simulink model "traction_control_simulink"  (R2020b)
settings: Solver=VariableStepAuto  StartTime=0.0  StopTime=3  RelTol=1e-3
values from neighbouring files (symbols this model uses):
  N = 4    [run_simulation.m]
  Ts = 2e-3    (= 0.002)    [run_simulation.m]
  x0 = [1.4; 4.4]    [run_simulation.m]
libraries: pid_lib x1
settings Model: Creator=LAMES Workstation  LastModifiedBy=LAMES Workstation

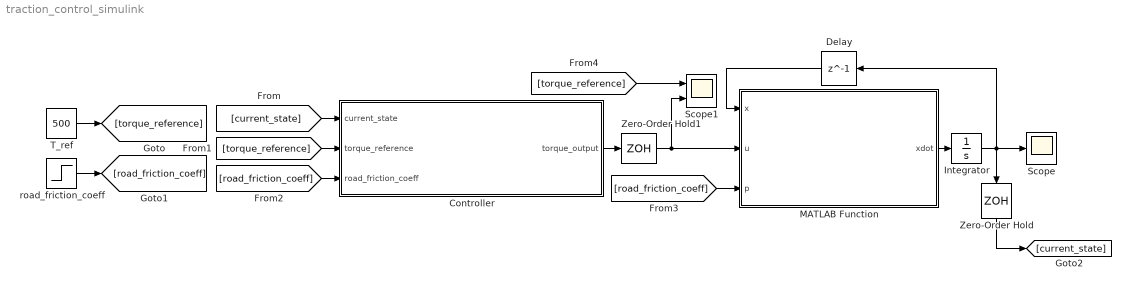
== system traction_control_simulink ==
  Controller : Subsystem  Variant=on
  Delay : Delay  DelayLength=1  InitialCondition=x0
  Integrator : Integrator  InitialCondition=x0
  MATLAB Function : MATLAB Function  TreatAsAtomicUnit=on
  Scope : Scope
  Scope1 : Scope  NumInputPorts=2
  T_ref : Constant  Value=500  SampleTime=Ts
  Zero-Order Hold : ZeroOrderHold  SampleTime=Ts
  Zero-Order Hold1 : ZeroOrderHold  SampleTime=Ts/100
  road_friction_coeff : Step  Time=0.5  Before=0.15  After=0.05  SampleTime=Ts
  wires:
  [road_friction_coeff] -> MATLAB Function/3(p)
  Delay/1 -> MATLAB Function/1(x)
  MATLAB Function/1(xdot) -> Integrator/1
  Zero-Order Hold/1 -> [current_state]
  Zero-Order Hold1/1 -> Scope1/2, MATLAB Function/2(u)
  Integrator/1 -> Zero-Order Hold/1, Scope/1, Delay/1
  T_ref/1 -> [torque_reference]
  road_friction_coeff/1 -> [road_friction_coeff]
  [current_state] -> Controller/1(current_state)
  Controller/1(torque_output) -> Zero-Order Hold1/1
  [torque_reference] -> Controller/2(torque_reference)
  [road_friction_coeff] -> Controller/3(road_friction_coeff)
  [torque_reference] -> Scope1/1

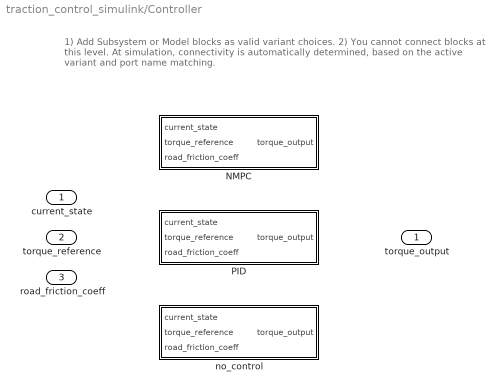
== system traction_control_simulink/Controller ==
  note: 1) Add Subsystem or Model blocks as valid variant choices.
      | 2) You cannot connect blocks at this level. At simulation, connectivity is automatically
      | determined, based on the active variant and port name matching.
  current_state : Inport
  torque_reference : Inport  Port=2
  road_friction_coeff : Inport  Port=3
  NMPC : Subsystem  VariantControl=controller_type == 1
  PID : Subsystem  VariantControl=controller_type == 3
  no_control : Subsystem  VariantControl=controller_type == 0
  torque_output : Outport

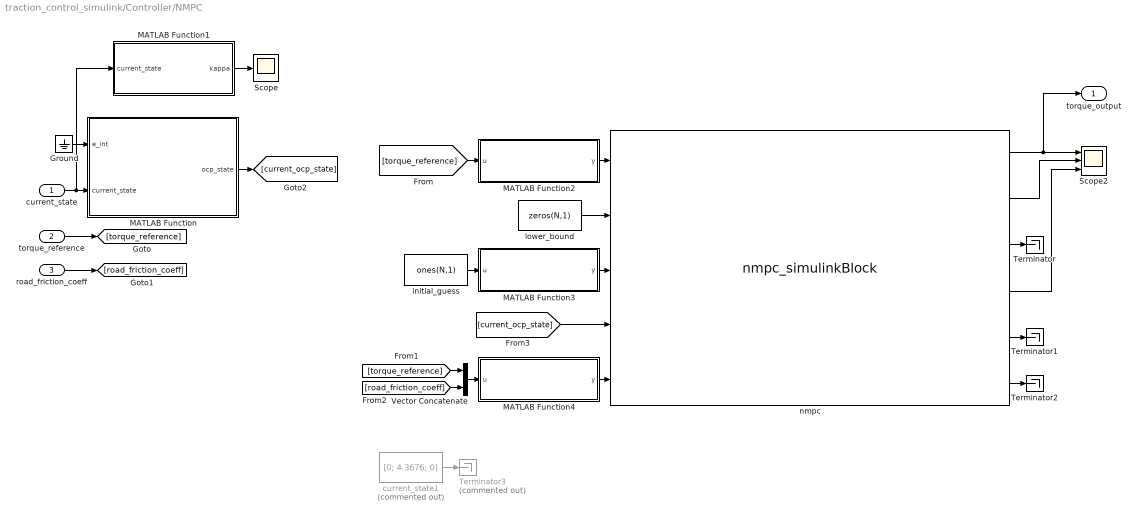
== system traction_control_simulink/Controller/NMPC ==
  current_state : Inport
  torque_reference : Inport  Port=2
  road_friction_coeff : Inport  Port=3
  Ground : Ground
  MATLAB Function : MATLAB Function  TreatAsAtomicUnit=on
  MATLAB Function1 : MATLAB Function  TreatAsAtomicUnit=on
  MATLAB Function2 : MATLAB Function  TreatAsAtomicUnit=on
  MATLAB Function3 : MATLAB Function  TreatAsAtomicUnit=on
  MATLAB Function4 : MATLAB Function  TreatAsAtomicUnit=on
  Scope : Scope
  Scope2 : Scope  NumInputPorts=3
  Terminator : Terminator
  Terminator1 : Terminator
  Terminator2 : Terminator
  Terminator3 : Terminator  Commented=on
  Vector Concatenate : Concatenate
  current_state1 : Constant  Commented=on  Value=[0; 4.3676; 0]  SampleTime=Ts
  initial_guess : Constant  Value=ones(N,1)  SampleTime=Ts
  lower_bound : Constant  Value=zeros(N,1)  SampleTime=Ts
  nmpc : S-Function  FunctionName=nmpc_simulinkBlock  SFunctionModules=nmpc nmpc_simulinkBlock  SFunctionDeploymentMode=off  EnableBusSupport=off  mask(nmpc_simulinkBlock){}
      mask help:
      | ---- Simulink block encapsulating your customized solver nmpc ----
      |
      | nmpc : A fast customized optimization solver.
      |
      | Copyright (C) 2013-2023 EMBOTECH AG [info@embotech.com]. All rights reserved.
      |
      |
      | This program is distributed in the hope that it will be useful.
      | EMBOTECH makes NO WARRANTIES with respect to the use of the software
      | without even the implied warranty of MERCHANTABILITY or FITNESS FOR A
      | PARTICULAR PURPOSE.
      |
      | EMBOTECH shall not have any liability for any damage arising from the use
      | of the software.
      |
      | This Agreement shall exclusively be governed by and interpreted in
      | accordance with the laws of Switzerland, excluding its principles
      | of conflict of laws. The Courts of Zurich-City shall have exclusive
      | jurisdiction in case of any dispute.
      mask Help:
      | nmpc_simulinkBlock provides an easy Simulink interface for simulating your customized solver.
      | 
      | OUTPUTS = nmpc(INPUTS) solves an optimization problem where:
      | 
      | INPUTS:
      |  - hu - matrix of size [4x1]
      |    - hl - matrix of size [4x1]
      |    - x0 - matrix of size [16x1]
      |    - xinit - matrix of size [3x1]
      |    - all_parameters - matrix of size [8x1]
      | 
      | OUTPUTS:
      |  - u0 - scalar
      |    - exitflag - scalar: (1) Optimal solution has been found (subject to desired accuracy); (0) Maximum number of interior point iterations reached; (-7) Line search could not progress
      |    - iterations - iteration number
      |    - solve_time - total solve time
      |    - primal_obj - primal objective
      |    - solver_id - solver ID of FORCESPRO solver
      | 
      |  For more information, see https://forces.embotech.com/Documentation/simulink_interface/index.html
      mask Display:
      | port_label('input', 1, 'hu')
      |   port_label('input', 2, 'hl')
      |   port_label('input', 3, 'x0')
      |   port_label('input', 4, 'xinit')
      |   port_label('input', 5, 'all_parameters')
      |   port_label('output', 1, 'u0')
      |   port_label('output', 2, 'exitflag')
      |   port_label('output', 3, 'iterations')
      |   port_label('output', 4, 'solve_time')
      |   port_label('output', 5, 'primal_obj')
      |   port_label('output', 6, 'solver_id')
      |   if( exist('FORCES_PRO_Logo.jpg','file') ), image(imread('FORCES_PRO_Logo.jpg'),'center','on'); elseif( exist(['interface',filesep,'FORCES_PRO_Logo.jpg'],'file') ), image(imread(['interface',filesep,'FORCES_PRO_Logo.jpg']),'center','on'); elseif( exist(['nmpc',filesep,'interface',filesep,'FORCES_PRO_Logo.jpg'],'file') ), image(imread(['nmpc',filesep,'interface',filesep,'FORCES_PRO_Logo.jpg']),'center','on'); end
  torque_output : Outport
  wires:
  [current_ocp_state] -> nmpc/4
  initial_guess/1 -> MATLAB Function3/1(u)
  nmpc/3 -> Terminator/1
  nmpc/6 -> Terminator2/1
  nmpc/2 -> Scope2/2
  nmpc/1 -> torque_output/1, Scope2/1
  lower_bound/1 -> nmpc/2
  nmpc/4 -> Scope2/3
  [road_friction_coeff] -> Vector Concatenate/2
  Vector Concatenate/1 -> MATLAB Function4/1(u)
  [torque_reference] -> Vector Concatenate/1
  nmpc/5 -> Terminator1/1
  MATLAB Function2/1(y) -> nmpc/1
  [torque_reference] -> MATLAB Function2/1(u)
  MATLAB Function3/1(y) -> nmpc/3
  MATLAB Function4/1(y) -> nmpc/5
  torque_reference/1 -> [torque_reference]
  road_friction_coeff/1 -> [road_friction_coeff]
  current_state/1 -> MATLAB Function1/1(current_state), MATLAB Function/2(current_state)
  MATLAB Function/1(ocp_state) -> [current_ocp_state]
  Ground/1 -> MATLAB Function/1(e_int)
  current_state1/1 -> Terminator3/1
  MATLAB Function1/1(kappa) -> Scope/1

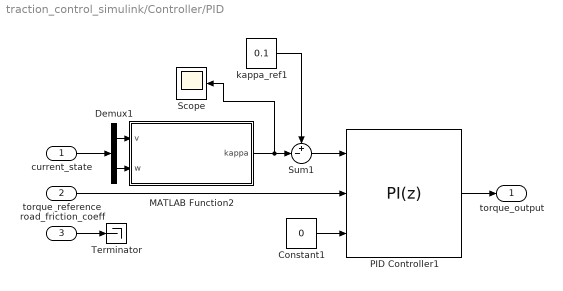
== system traction_control_simulink/Controller/PID ==
  current_state : Inport
  torque_reference : Inport  Port=2
  road_friction_coeff : Inport  Port=3
  Constant1 : Constant  Value=0  SampleTime=Ts
  Demux1 : Demux  Outputs=2
  MATLAB Function2 : MATLAB Function  TreatAsAtomicUnit=on
  PID Controller1 : pid_lib/PID Controller  Controller=PI  Form=Parallel  TimeDomain=Discrete-time  UseExternalTs=off  SampleTime=-1  IntegratorMethod=Forward Euler  FilterMethod=Forward Euler  ControllerParametersSource=internal  P=3500  I=40000  D=0  UseFilter=on  N=100  TunerSelectOption=Transfer Function Based (PID Tuner App)  InitialConditionSource=internal  InitialConditionForIntegrator=0  InitialConditionForFilter=0  DifferentiatorICPrevScaledInput=0  ExternalReset=none  TrackingMode=off  Kt=1  LimitOutput=on  SatLimitsSource=external  UpperSaturationLimit=500  LowerSaturationLimit=0  LinearizeAsGain=on  AntiWindupMode=clamping  Kb=1  POutMin=[]  POutMax=[]  IOutMin=[]  IOutMax=[]  DOutMin=[]  DOutMax=[]  NOutMin=[]  NOutMax=[]  SumOutMin=[]  SumOutMax=[]  SaturationOutMin=[]  SaturationOutMax=[]  PParamMin=[]  PParamMax=[]  IParamMin=[]  IParamMax=[]  DParamMin=[]  DParamMax=[]  NParamMin=[]  NParamMax=[]  KbParamMin=[]  KbParamMax=[]  KtParamMin=[]  KtParamMax=[]  KbOutMin=[]  KbOutMax=[]  KtOutMin=[]  KtOutMax=[]  IntegratorOutMin=[]  IntegratorOutMax=[]  FilterOutMin=[]  FilterOutMax=[]  SumI1OutMin=[]  SumI1OutMax=[]  SumI2OutMin=[]  SumI2OutMax=[]  SumI3OutMin=[]  SumI3OutMax=[]  SumI4OutMin=[]  SumI4OutMax=[]  SumDOutMin=[]  SumDOutMax=[]  DifferentiatorOutMin=[]  DifferentiatorOutMax=[]  FilterDiffOutCoefMin=[]  FilterDiffOutCoefMax=[]  ReciprocalOutMin=[]  ReciprocalOutMax=[]  SumDenOutMin=[]  SumDenOutMax=[]  SumNumOutMin=[]  SumNumOutMax=[]  DivideOutMin=[]  DivideOutMax=[]  UdiffTsProdOutMin=[]  UdiffTsProdOutMax=[]  NTsProdOutMin=[]  NTsProdOutMax=[]  UintegralTsProdOutMin=[]  UintegralTsProdOutMax=[]  UngainTsProdOutMin=[]  UngainTsProdOutMax=[]  IntegratorContinuousStateAttributes=''  IntegratorStateMustResolveToSignalObject=off  IntegratorRTWStateStorageClass=Auto  FilterContinuousStateAttributes=''  FilterStateMustResolveToSignalObject=off  FilterRTWStateStorageClass=Auto  ParallelPVariant=InternalParameters  IdealPVariant=Disabled  IVariant=InternalParameters  DVariant=Disabled  IntegratorVariant=Discrete  SatVariant=External  AWVariant=DiscClampingParallel  PCopyVariant=Disabled  TRVariant=Disabled  FdbkBlocksVariant=Forward  IdealPFdbkVariant=Disabled  SatFdbkVariant=Disabled  DerivativeFilterVariant=Disabled  NVariant=Disabled  NCopyVariant=Disabled_SignalSpec  FilterICVariant=Disabled  IntegratorICVariant=InternalICs  ExternalResetVariant=Disabled  TRSumVariant=Passthrough  SumFdbkVariant=Disabled  SumVariant=Sum_PI  TsampFilterVariant=InternalTs  TsampNgainVariant=Passthrough  TsampIntegralVariant=Passthrough  ExternalSaturationOutDataTypeStr=Inherit: Same as second input
  Scope : Scope
  Sum1 : Sum  Inputs=+-|
  Terminator : Terminator
  kappa_ref1 : Constant  Value=0.1  SampleTime=Ts
  torque_output : Outport
  wires:
  PID Controller1/1 -> torque_output/1
  torque_reference/1 -> PID Controller1/2
  road_friction_coeff/1 -> Terminator/1
  kappa_ref1/1 -> Sum1/1
  Demux1/1 -> MATLAB Function2/1(v)
  Demux1/2 -> MATLAB Function2/2(w)
  current_state/1 -> Demux1/1
  MATLAB Function2/1(kappa) -> Scope/1, Sum1/2
  Sum1/1 -> PID Controller1/1
  Constant1/1 -> PID Controller1/3

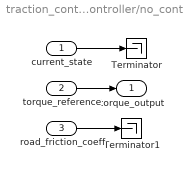
== system traction_control_simulink/Controller/no_control ==
  current_state : Inport
  torque_reference : Inport  Port=2
  road_friction_coeff : Inport  Port=3
  Terminator : Terminator
  Terminator1 : Terminator
  torque_output : Outport
  wires:
  current_state/1 -> Terminator/1
  road_friction_coeff/1 -> Terminator1/1
  torque_reference/1 -> torque_output/1

== matlab function traction_control_simulink/MATLAB Function ==
  data: x input; u input; xdot output; p input
function xdot = simulation_model_ode(x,u,p)
% TODO: find realistic motor torque limit and driving situation for slip
% wet asphalt? (Fig. 4 in https://ieeexplore.ieee.org/document/6043067)

% system dimensions
% nx = 2;  % vehicle speed, wheel speed
% nu = 1;  % wheel torque

% system parameters
m = 1600/4;     % [kg] quarter car mass
g = 9.81;       % [m/s^2] gravity constant
R = 0.318;      % [m] wheel radius
Jw = 1.22;      % [kg*m^2] moment of inertia for one wheel and half-axle
T_max = 500;    % [Nm] maximum motor torque
mu_x = p(1);    % [-] tire-road friction coefficient

% tire model coefficients Fx=mu_x*Fz*D*sin(C*arctan(B*kappa))
% Carmaker MF_205_60R15_V91.tir
D = 1.2005;
C = 1.4010;
B = 17.1571;

% Saab?
% D = 1.2069;
% C = 1.35;
% K = 30;
% B = K/(C*D);

% state and input variables
v = x(1);           % longitudinal speed of the vehicle [m/s]
w = x(2);           % rotational speed of the wheel [rad/s]
T = min(u,T_max);   % motor torque acting on the wheel [Nm]

% dynamics
Fz = m*g;
kappa = (w*R-v)/(w*R);
Fx = mu_x * Fz * D*sin(C*atan(B*kappa));
vdot = Fx/m;
wdot = 1/Jw * (T-Fx*R);

xdot = [vdot;wdot];
end

== matlab function traction_control_simulink/Controller/NMPC/MATLAB Function2 ==
  data: u input; y output; N parameter
function y = repeat_elements(u, N)
    y = repmat(u,N,1);
end

== matlab function traction_control_simulink/Controller/NMPC/MATLAB Function3 ==
  data: u input; y output; N parameter
function y = repeat_elements(u, N)
    y = repmat(u,N,1);
end

== matlab function traction_control_simulink/Controller/NMPC/MATLAB Function4 ==
  data: u input; y output; N parameter
function y = repeat_elements(u, N)
    y = repmat(u,N,1);
end

== matlab function traction_control_simulink/Controller/NMPC/MATLAB Function1 ==
  data: current_state input; kappa output; R parameter
function kappa = calculate_slip(current_state,R)
    v = current_state(1);
    w = current_state(2);
    kappa = 1-v/(w*R);
end

== matlab function traction_control_simulink/Controller/PID/MATLAB Function2 ==
  data: v input; kappa output; w input; R parameter
function kappa = calculate_slip(v,w,R)
    kappa = 1-v/(w*R);
end

== matlab function traction_control_simulink/Controller/NMPC/MATLAB Function ==
  data: e_int input; current_state input; ocp_state output; R parameter
function ocp_state = create_ocp_state(e_int,current_state, R)
    v = current_state(1);
    w = current_state(2);
    ocp_state = [w*R-v; w; e_int];
end
